simulink model "threephase_rlc_mm"  (R2014a)
settings: Solver=ode45  StartTime=0.0  StopTime=10  MaxStep=1e-3  RelTol=1e-3
libraries: powerlib x7
settings Model: Creator=cosorio  LastModifiedBy=cosorio

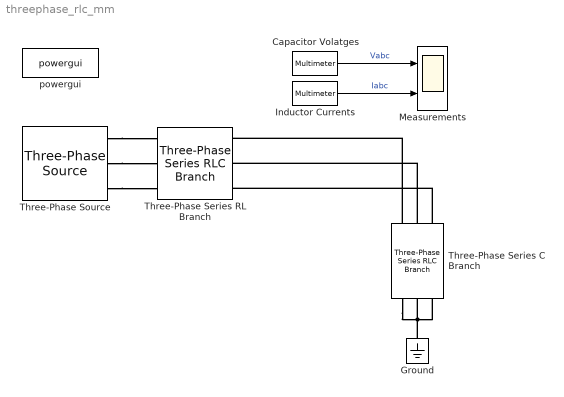
== system threephase_rlc_mm ==
  Capacitor Volatges : powerlib/Measurements/Multimeter  PhasorSimulation=off  OutputType=Complex  sel=[1 2 3]  L=6  Gain=[1 1 1]  yselected={'Ub1: Three-Phase Series C Branch','Ub2: Three-Phase Series C Branch','Ub3: Three-Phase Series C Branch'};  PSBOutputType=1  PSBequivalent=0  AxesSetting=[0,0.1,-100,100]  Display=0  SavedBlockNames=-11
  Ground : powerlib/Elements/Ground  LConnTagsString=a
  Inductor Currents : powerlib/Measurements/Multimeter  PhasorSimulation=off  OutputType=Complex  sel=[4 5 6]  L=6  Gain=[1 1 1]  yselected={'Ib1: Three-Phase Series RL Branch','Ib2: Three-Phase Series RL Branch','Ib3: Three-Phase Series RL Branch'};  PSBOutputType=1  PSBequivalent=0  AxesSetting=[0,0.1,-100,100]  Display=0  SavedBlockNames=-11
  Measurements : Scope  NumInputPorts=2
      settings: YMin=-40000~-10  YMax=40000~10
  Three-Phase Series C Branch : powerlib/Elements/Three-Phase Series RLC Branch  LConnTagsString=A|B|C  RConnTagsString=A|B|C  BranchType=C  Resistance=1  Inductance=1e-3  Capacitance=1e-6  Measurements=Branch voltages
  Three-Phase Series RL Branch : powerlib/Elements/Three-Phase Series RLC Branch  LConnTagsString=A|B|C  RConnTagsString=A|B|C  BranchType=RL  Resistance=1  Inductance=1e-3  Capacitance=1e-6  Measurements=Branch currents
  Three-Phase Source : powerlib/Electrical Sources/Three-Phase Source  Voltage=25e3  PhaseAngle=0  Frequency=60  InternalConnection=Yg  SpecifyImpedance=on  Resistance=0.8929  Inductance=16.58e-3  ShortCircuitLevel=100e6  BaseVoltage=25e3  XRratio=7  BusType=swing  Pref=0  Qref=0  Qmin=-inf  Qmax=inf
  powergui : powerlib/powergui  Priority=1  SimulationMode=Continuous  SolverType=Tustin  SampleTime=50e-6  frequency=60  SPID=off  DisableSnubberDevices=off  DisableRonSwitches=off  DisableVfSwitches=off  SwTol=0  Interpol=off  DisplayEquations=off  Ts=0  methode=off  frequencyindice=60  Pbase=100e6  ErrMax=1e-4  Iterations=50  UnitsV=kV  UnitsW=MW  FunctionMessages=off  echomessages=off  HookPort=off  EnableUseOfTLC=off  x0status=blocks  RestoreLinks=warning  ResistiveCurrentMeasurement=off  Frange=[0:2:500]  Ylog=off  Xlog=on  ShowGrid=off  save=off  variable=ZData  structure=0  ZoomFFT=off  StartTime=0.0  cycles=1  DisplayStyle=1  fundamental=60  FreqAxis=off  MaxFrequency=1000  frequencyindicesteady=1  RmsSteady=1  display=off
  wires:
  Capacitor Volatges/1 -> Measurements/1  "Vabc"
  Inductor Currents/1 -> Measurements/2  "Iabc"
  connections:
  Three-Phase Source/RConn1 -- Three-Phase Series RL Branch/LConn1
  Three-Phase Source/RConn2 -- Three-Phase Series RL Branch/LConn2
  Three-Phase Source/RConn3 -- Three-Phase Series RL Branch/LConn3
  Three-Phase Series C Branch/LConn1 -- Three-Phase Series RL Branch/RConn1
  Three-Phase Series C Branch/LConn2 -- Three-Phase Series RL Branch/RConn2
  Three-Phase Series C Branch/LConn3 -- Three-Phase Series RL Branch/RConn3
  Ground/LConn1 -- Three-Phase Series C Branch/RConn3 -- Three-Phase Series C Branch/RConn1 -- Three-Phase Series C Branch/RConn2
